simulink model "ex_1"  (R2021a)
settings: Solver=VariableStepAuto  StartTime=0.0  StopTime=10  RelTol=1e-3
settings Model: Creator=HanO  LastModifiedBy=HanO

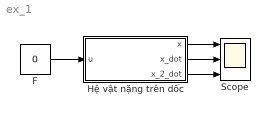
== system ex_1 ==
  F : Constant  Value=0
  Hệ vật nặng trên dốc : Subsystem  mask{m=3, g=9.81, alpha=pi/6, x0=0}
      mask prompts: m "Khối lượng vật nặng m [kg]"; g "Gia tốc trọng trường g [m/s2]"; alpha "Độ nghiêng con dốc alpha [rad]"; x0 "Vị trí đầu của vật nặng"
  Scope : Scope  NumInputPorts=3
  wires:
  F/1 -> Hệ vật nặng trên dốc/1(u)
  Hệ vật nặng trên dốc/1(x) -> Scope/1
  Hệ vật nặng trên dốc/2(x_dot) -> Scope/2
  Hệ vật nặng trên dốc/3(x_2_dot) -> Scope/3

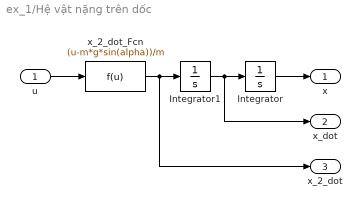
== system ex_1/Hệ vật nặng trên dốc ==
  u : Inport
  Integrator : Integrator  InitialCondition=x0
  Integrator1 : Integrator
  x_2_dot_Fcn : Fcn  Expr=(u-m*g*sin(alpha))/m
  x : Outport
  x_dot : Outport  Port=2
  x_2_dot : Outport  Port=3
  wires:
  Integrator1/1 -> x_dot/1, Integrator/1
  Integrator/1 -> x/1
  x_2_dot_Fcn/1 -> x_2_dot/1, Integrator1/1
  u/1 -> x_2_dot_Fcn/1
